simulink library "INP_IMU_ManOver2"  (R2024b)
settings: Solver=VariableStepAuto  StartTime=0.0  StopTime=10.0  RelTol=1e-3
undefined symbols (not defined in the file): INP_IMU_p_ALatVehLoLim_mps2, INP_IMU_p_ALatVehMan_mps2, INP_IMU_p_ALatVehUpLim_mps2, INP_IMU_p_ALgtVehLoLim_mps2, INP_IMU_p_ALgtVehMan_mps2, INP_IMU_p_ALgtVehUpLim_mps2, INP_IMU_p_AVertVehLoLim_mps2, INP_IMU_p_AVertVehMan_mps2, INP_IMU_p_AVertVehUpLim_mps2, INP_IMU_p_SwtALatVehMan_na, INP_IMU_p_SwtALgtVehMan_na, INP_IMU_p_SwtAVertVehMan_na
libraries: simulink x3
settings Model: Creator=blatak  LastModifiedBy=jmbsp
settings RTWCC: GPUComputeCapability=3.5

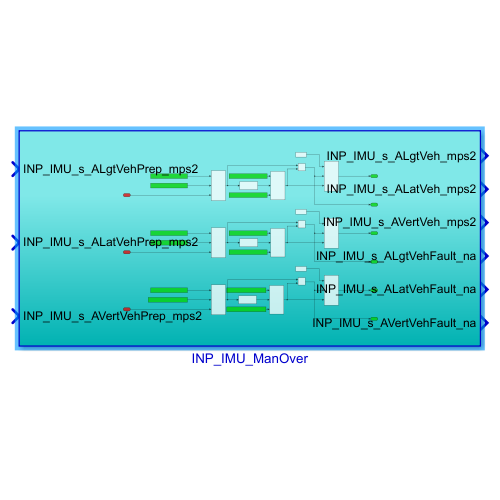
[thumbnail: Simulink's stored preview of the top-level diagram]
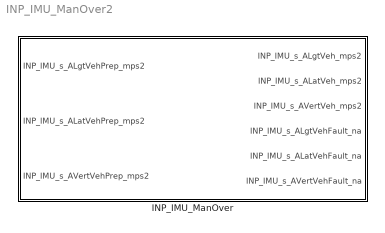
== system INP_IMU_ManOver2 ==
  INP_IMU_ManOver : Subsystem  Description=Manual override of measured value (some default value replaces the measured one) and saturation

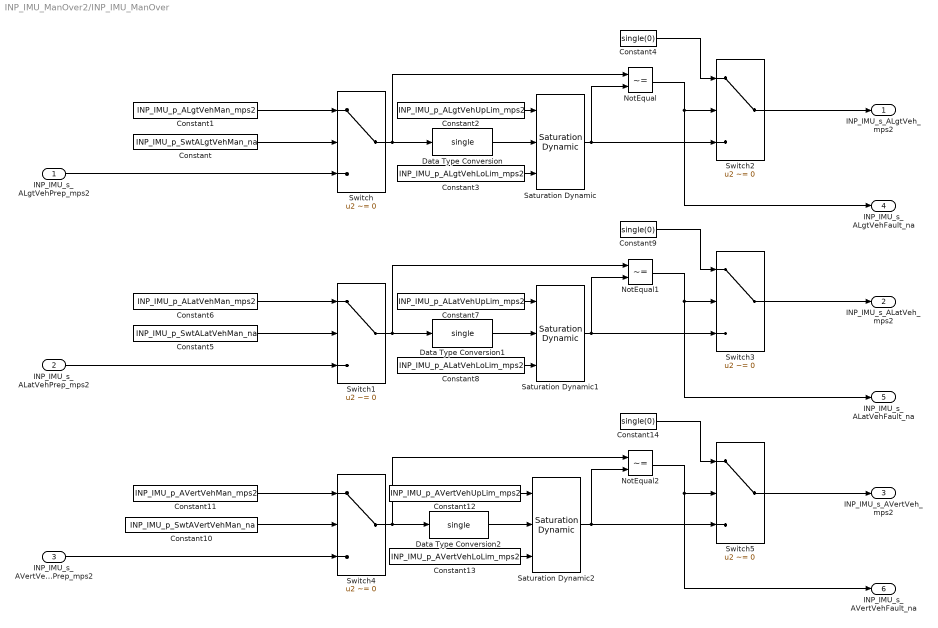
== system INP_IMU_ManOver2/INP_IMU_ManOver ==
  INP_IMU_s_ALgtVehPrep_mps2 : Inport  Description=IMU Prep Longitudinal acceleration - prepared value - scale, offset, filtering
  INP_IMU_s_ALatVehPrep_mps2 : Inport  Description=IMU Prep Lateral acceleration - prepared value - scale, offset, filtering  Port=2
  INP_IMU_s_AVertVehPrep_mps2 : Inport  Description=IMU Prep Vertical acceleration - prepared value - scale, offset, filtering  Port=3
  Constant : Constant  Description=|  Value=INP_IMU_p_SwtALgtVehMan_na
      | Switch for manual override of the longitudinal acceleration value, if 1 instead the measured 
      | value the INP_IMU_p_ALgtVehMan_mps2 is used
  Constant1 : Constant  Description=|  Value=INP_IMU_p_ALgtVehMan_mps2
      | Value for longitudinal acceleration, which is used if the INP_IMU_p_SwtAXxxVehMan_na
      | is set to 1 instead of the measured value
  Constant10 : Constant  Description=|  Value=INP_IMU_p_SwtAVertVehMan_na
      | Switch for manual override of the vertical acceleration value, if 1 instead the measured 
      | value the INP_IMU_p_ALgtVehMan_mps2 is used
  Constant11 : Constant  Description=|  Value=INP_IMU_p_AVertVehMan_mps2
      | Value for vertical acceleration, which is used if the INP_IMU_p_SwtAXxxVehMan_na
      | is set to 1 instead of the measured value
  Constant12 : Constant  Description=Upper saturation limit for vertical acceleration  Value=INP_IMU_p_AVertVehUpLim_mps2
  Constant13 : Constant  Description=Lower saturation limit for vertical acceleration  Value=INP_IMU_p_AVertVehLoLim_mps2
  Constant14 : Constant  Value=single(0)
  Constant2 : Constant  Description=Upper saturation limit for longitudinal acceleration  Value=INP_IMU_p_ALgtVehUpLim_mps2
  Constant3 : Constant  Description=Lower saturation limit for longitudinal acceleration  Value=INP_IMU_p_ALgtVehLoLim_mps2
  Constant4 : Constant  Value=single(0)
  Constant5 : Constant  Description=|  Value=INP_IMU_p_SwtALatVehMan_na
      | Switch for manual override of the lateral acceleration value, if 1 instead the measured 
      | value the INP_IMU_p_ALgtVehMan_mps2 is used
  Constant6 : Constant  Description=|  Value=INP_IMU_p_ALatVehMan_mps2
      | Value for lateral acceleration, which is used if the INP_IMU_p_SwtAXxxVehMan_na
      | is set to 1 instead of the measured value
  Constant7 : Constant  Description=Upper saturation limit for lateral acceleration  Value=INP_IMU_p_ALatVehUpLim_mps2
  Constant8 : Constant  Description=Lower saturation limit for lateral acceleration  Value=INP_IMU_p_ALatVehLoLim_mps2
  Constant9 : Constant  Value=single(0)
  Data Type Conversion : DataTypeConversion  OutDataTypeStr=single  SaturateOnIntegerOverflow=off  RndMeth=Floor
  Data Type Conversion1 : DataTypeConversion  OutDataTypeStr=single  SaturateOnIntegerOverflow=off  RndMeth=Floor
  Data Type Conversion2 : DataTypeConversion  OutDataTypeStr=single  SaturateOnIntegerOverflow=off  RndMeth=Floor
  NotEqual : RelationalOperator  Operator=~=  OutDataTypeStr=boolean  RndMeth=Simplest  InputSameDT=off
  NotEqual1 : RelationalOperator  Operator=~=  OutDataTypeStr=boolean  RndMeth=Simplest  InputSameDT=off
  NotEqual2 : RelationalOperator  Operator=~=  OutDataTypeStr=boolean  RndMeth=Simplest  InputSameDT=off
  Saturation Dynamic : simulink/Discontinuities/Saturation Dynamic  OutMin=[]  OutMax=[]  OutDataTypeStr=Inherit: Same as second input  OutDataType=fixdt(1, 16)  OutScaling=2^-10  DoSatur=off
  Saturation Dynamic1 : simulink/Discontinuities/Saturation Dynamic  OutMin=[]  OutMax=[]  OutDataTypeStr=Inherit: Same as second input  OutDataType=fixdt(1, 16)  OutScaling=2^-10  DoSatur=off
  Saturation Dynamic2 : simulink/Discontinuities/Saturation Dynamic  OutMin=[]  OutMax=[]  OutDataTypeStr=Inherit: Same as second input  OutDataType=fixdt(1, 16)  OutScaling=2^-10  DoSatur=off
  Switch{,1..5} (6 alike) : Switch  Criteria=u2 ~= 0  SaturateOnIntegerOverflow=off  InputSameDT=off
  INP_IMU_s_ALgtVeh_mps2 : Outport  Description=INP IMU Vehicle longitudinal acceleration - manual override, saturation
  INP_IMU_s_ALatVeh_mps2 : Outport  Description=INP IMU Vehicle lateral acceleration - manual override, saturation  Port=2
  INP_IMU_s_AVertVeh_mps2 : Outport  Description=INP IMU Vehicle vertical acceleration - manual override, saturation  Port=3
  INP_IMU_s_ALgtVehFault_na : Outport  Port=4
  INP_IMU_s_ALatVehFault_na : Outport  Port=5
  INP_IMU_s_AVertVehFault_na : Outport  Port=6
  wires:
  NotEqual2/1 -> INP_IMU_s_AVertVehFault_na/1, Switch5/2
  Constant2/1 -> Saturation Dynamic/1
  INP_IMU_s_AVertVehPrep_mps2/1 -> Switch4/3
  Constant7/1 -> Saturation Dynamic1/1
  NotEqual1/1 -> INP_IMU_s_ALatVehFault_na/1, Switch3/2
  Constant8/1 -> Saturation Dynamic1/3
  Saturation Dynamic2/1 -> Switch5/3, NotEqual2/2
  INP_IMU_s_ALatVehPrep_mps2/1 -> Switch1/3
  Constant4/1 -> Switch2/1
  Switch1/1 -> NotEqual1/1, Data Type Conversion1/1
  Constant/1 -> Switch/2
  Saturation Dynamic/1 -> Switch2/3, NotEqual/2
  Switch/1 -> NotEqual/1, Data Type Conversion/1
  Constant10/1 -> Switch4/2
  INP_IMU_s_ALgtVehPrep_mps2/1 -> Switch/3
  Constant11/1 -> Switch4/1
  Constant13/1 -> Saturation Dynamic2/3
  Constant3/1 -> Saturation Dynamic/3
  Constant14/1 -> Switch5/1
  Saturation Dynamic1/1 -> Switch3/3, NotEqual1/2
  Constant5/1 -> Switch1/2
  Switch2/1 -> INP_IMU_s_ALgtVeh_mps2/1
  Constant6/1 -> Switch1/1
  Switch4/1 -> NotEqual2/1, Data Type Conversion2/1
  NotEqual/1 -> INP_IMU_s_ALgtVehFault_na/1, Switch2/2
  Switch3/1 -> INP_IMU_s_ALatVeh_mps2/1
  Constant1/1 -> Switch/1
  Switch5/1 -> INP_IMU_s_AVertVeh_mps2/1
  Constant9/1 -> Switch3/1
  Constant12/1 -> Saturation Dynamic2/1
  Data Type Conversion/1 -> Saturation Dynamic/2
  Data Type Conversion1/1 -> Saturation Dynamic1/2
  Data Type Conversion2/1 -> Saturation Dynamic2/2
